simulink model "HIL"  (R2023b)
settings: Solver=VariableStepAuto  StartTime=0.0  StopTime=10  FixedStep=0.01  RelTol=1e-3
values from neighbouring files (symbols this model uses):
  K = Z/P    [LMI.m]    (also in Workspace.mat = 8.82782218537; model_simulation.m = lqr(A,B,Q,R))
undefined symbols (not defined in the file or in its folder): CR, LF
libraries: instrumentseriallib x3
settings Model: Creator=petri  LastModifiedBy=petri

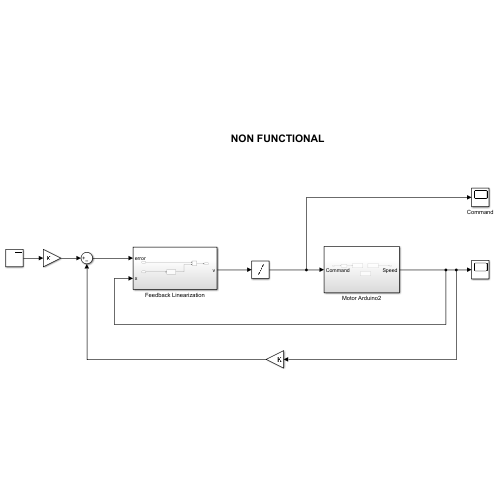
[thumbnail: Simulink's stored preview of the top-level diagram]
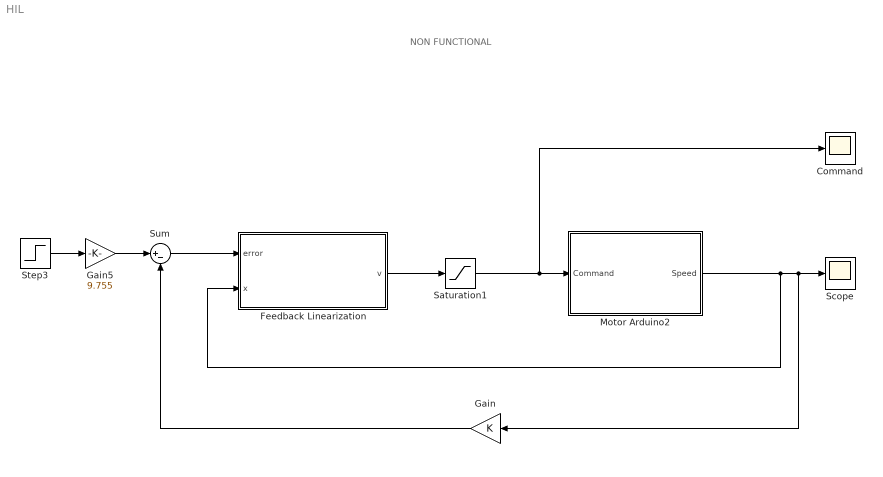
== system HIL ==
  note: NON FUNCTIONAL
  Command : Scope
  Feedback Linearization : Subsystem
  Gain : Gain  Gain=K
  Gain5 : Gain  Gain=9.755
  Motor Arduino2 : Subsystem
  Saturation1 : Saturate  UpperLimit=0.3  LowerLimit=0
  Scope : Scope
  Step3 : Step  Time=0  After=98  SampleTime=0
  Sum : Sum  Inputs=|+-
  wires:
  Sum/1 -> Feedback Linearization/1(error)
  Gain/1 -> Sum/2
  Step3/1 -> Gain5/1
  Gain5/1 -> Sum/1
  Feedback Linearization/1(v) -> Saturation1/1
  Saturation1/1 -> Motor Arduino2/1(Command), Command/1
  Motor Arduino2/1(Speed) -> Feedback Linearization/2(x), Gain/1, Scope/1

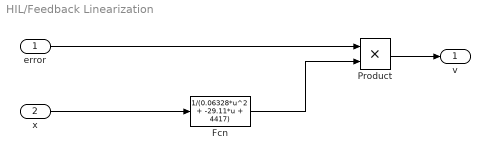
== system HIL/Feedback Linearization ==
  error : Inport
  x : Inport  Port=2
  Fcn : Fcn  Expr=1/(0.06328*u^2 + -29.11*u + 4417)
  Product : Product
  v : Outport
  wires:
  Product/1 -> v/1
  Fcn/1 -> Product/2
  error/1 -> Product/1
  x/1 -> Fcn/1

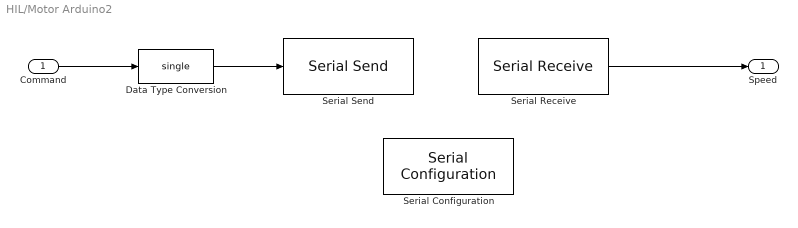
== system HIL/Motor Arduino2 ==
  Command : Inport
  Data Type Conversion : DataTypeConversion  OutDataTypeStr=single  SaturateOnIntegerOverflow=off  RndMeth=Floor
  Serial Configuration : instrumentseriallib/Serial Configuration  Priority=-200000  PortSel=COM3  Port=COM3  ComPort=COM3  BaudRate=115200  DataBits=8  Parity=none  StopBits=1  ByteOrder=little-endian  FlowControl=none  Timeout=10  SimulateUsing=Interpreted execution  BlockInModel=on  aMode=1
  Serial Receive : instrumentseriallib/Serial Receive  Priority=1  PortSel=COM3  Port=COM3  ComPort=COM3  DataType=single  SaveDataType=uint8  ToggleHeader=off  Header=[]  ToggleTerminator=on  Terminator=CR/LF ('\r\n')  CustomTerminator=[]  InputFormat=Column major  ToggleDataSize=on  DataSize=[1 1]  EnableBlockingMode=on  ActionDataUnavailable=Output last received value  ActionWhenDataUnavailable=Output last received value  CustomValue=0  SampleTime=0.01  SimulateUsing=Interpreted execution  BlockInModel=on  aMode=1
  Serial Send : instrumentseriallib/Serial Send  Priority=1  PortSel=COM3  Port=COM3  ComPort=COM3  Header=[]  Terminator=CR/LF ('\r\n')  CustomTerminator=[]  EnableBlockingMode=on  SimulateUsing=Interpreted execution  BlockInModel=on  aMode=1
  Speed : Outport
  wires:
  Serial Receive/1 -> Speed/1
  Data Type Conversion/1 -> Serial Send/1
  Command/1 -> Data Type Conversion/1
